simulink model "PriceCalc"  (R2021b)
settings: Solver=VariableStepAuto  StartTime=0.0  StopTime=10.0  RelTol=1e-3
libraries: fuzblock x22, simulink x7
settings Model: Creator=nbelo  LastModifiedBy=nbelo
settings SolverCC: ZeroCrossControl=DisableAll

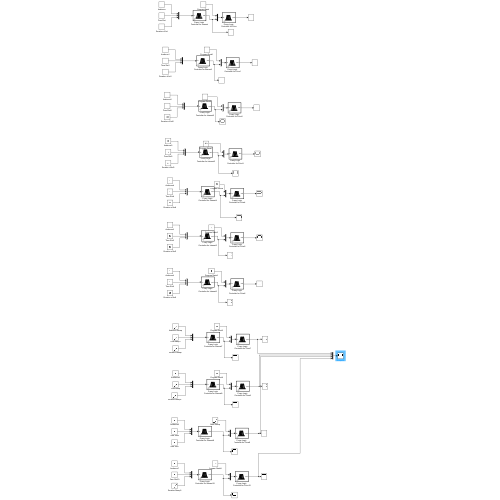
[thumbnail: Simulink's stored preview of the top-level diagram]
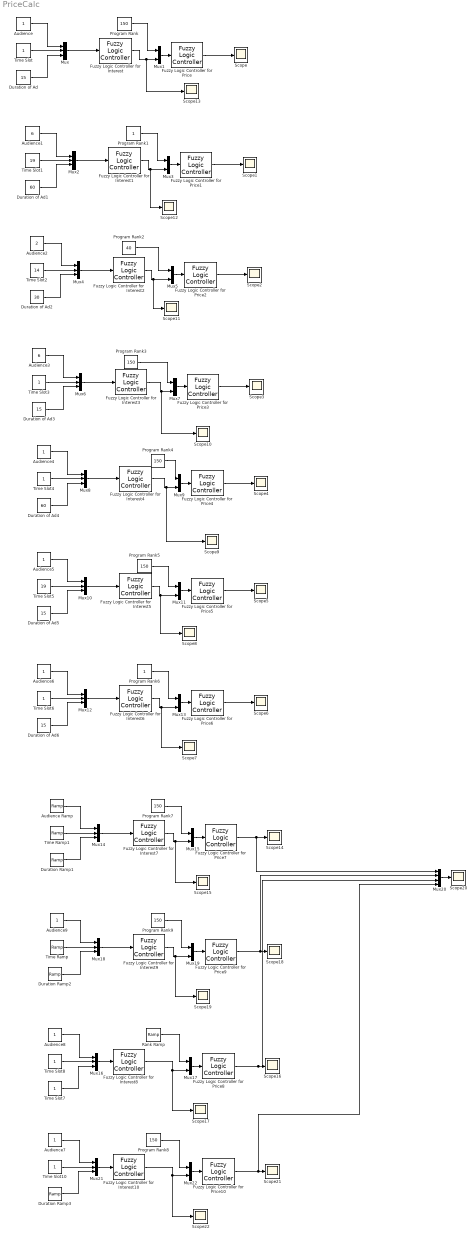
== system PriceCalc ==
  Audience{,4..9} (7 alike) : Constant
  Audience Ramp : simulink/Sources/Ramp  slope=.8  start=0  InitialOutput=0
  Audience1 : Constant  Value=6
  Audience2 : Constant  Value=2
  Audience3 : Constant  Value=6
  Duration Ramp1 : simulink/Sources/Ramp  slope=12  start=0  InitialOutput=0
  Duration Ramp2 : simulink/Sources/Ramp  slope=12  start=0  InitialOutput=0
  Duration Ramp3 : simulink/Sources/Ramp  slope=12  start=0  InitialOutput=0
  Duration of Ad{,3,5..6} (4 alike) : Constant  Value=15
  Duration of Ad1 : Constant  Value=60
  Duration of Ad2 : Constant  Value=30
  Duration of Ad4 : Constant  Value=60
  Fuzzy Logic Controller for Interest{,1..10} (11 alike) : fuzblock/Fuzzy Logic  Controller  FIS=Interest  OutputSampleNumber=101  DataType=double  FuzzifiedInputs=off  RuleFiringStrengths=off  RuleOutputs=off  AggregatedOutputs=off  SimulateUsing=Interpreted execution  OutOfRangeInputValueMessage=warning  NoRuleFiredMessage=warning  EmptyOutputFuzzySetMessage=warning
  Fuzzy Logic Controller for Price{,1..10} (11 alike) : fuzblock/Fuzzy Logic  Controller  FIS=Price  OutputSampleNumber=101  DataType=double  FuzzifiedInputs=off  RuleFiringStrengths=off  RuleOutputs=off  AggregatedOutputs=off  SimulateUsing=Interpreted execution  OutOfRangeInputValueMessage=warning  NoRuleFiredMessage=warning  EmptyOutputFuzzySetMessage=warning
  Mux{,2,4,6,8,10,12,14,16,18,21} (11 alike) : Mux  Inputs=3
  Mux{1,3,5,7,9,11,13,15,17,19,22} (11 alike) : Mux  Inputs=2
  Mux20 : Mux
  Program Rank{,3..5,7..9} (7 alike) : Constant  Value=150
  Program Rank1 : Constant
  Program Rank2 : Constant  Value=40
  Program Rank6 : Constant
  Rank Ramp : simulink/Sources/Ramp  slope=20  start=0  InitialOutput=0
  Scope{,1..22} (23 alike) : Scope
  Time Ramp : simulink/Sources/Ramp  slope=2.4  start=0  InitialOutput=0
  Time Ramp1 : simulink/Sources/Ramp  slope=2.4  start=0  InitialOutput=0
  Time Slot{,3..4,6..8,10} (7 alike) : Constant
  Time Slot1 : Constant  Value=19
  Time Slot2 : Constant  Value=14
  Time Slot5 : Constant  Value=19
  wires:
  Time Slot/1 -> Mux/2
  Audience/1 -> Mux/1
  Duration of Ad/1 -> Mux/3
  Mux/1 -> Fuzzy Logic Controller for Interest/1
  Mux1/1 -> Fuzzy Logic Controller for Price/1
  Fuzzy Logic Controller for Price/1 -> Scope/1
  Mux2/1 -> Fuzzy Logic Controller for Interest1/1
  Time Slot1/1 -> Mux2/2
  Audience1/1 -> Mux2/1
  Fuzzy Logic Controller for Price1/1 -> Scope1/1
  Mux3/1 -> Fuzzy Logic Controller for Price1/1
  Duration of Ad1/1 -> Mux2/3
  Mux4/1 -> Fuzzy Logic Controller for Interest2/1
  Time Slot2/1 -> Mux4/2
  Audience2/1 -> Mux4/1
  Fuzzy Logic Controller for Price2/1 -> Scope2/1
  Mux5/1 -> Fuzzy Logic Controller for Price2/1
  Duration of Ad2/1 -> Mux4/3
  Mux6/1 -> Fuzzy Logic Controller for Interest3/1
  Time Slot3/1 -> Mux6/2
  Audience3/1 -> Mux6/1
  Fuzzy Logic Controller for Price3/1 -> Scope3/1
  Mux7/1 -> Fuzzy Logic Controller for Price3/1
  Duration of Ad3/1 -> Mux6/3
  Mux8/1 -> Fuzzy Logic Controller for Interest4/1
  Time Slot4/1 -> Mux8/2
  Audience4/1 -> Mux8/1
  Fuzzy Logic Controller for Price4/1 -> Scope4/1
  Mux9/1 -> Fuzzy Logic Controller for Price4/1
  Duration of Ad4/1 -> Mux8/3
  Mux10/1 -> Fuzzy Logic Controller for Interest5/1
  Time Slot5/1 -> Mux10/2
  Audience5/1 -> Mux10/1
  Fuzzy Logic Controller for Price5/1 -> Scope5/1
  Mux11/1 -> Fuzzy Logic Controller for Price5/1
  Duration of Ad5/1 -> Mux10/3
  Mux12/1 -> Fuzzy Logic Controller for Interest6/1
  Time Slot6/1 -> Mux12/2
  Audience6/1 -> Mux12/1
  Fuzzy Logic Controller for Price6/1 -> Scope6/1
  Mux13/1 -> Fuzzy Logic Controller for Price6/1
  Duration of Ad6/1 -> Mux12/3
  Program Rank/1 -> Mux1/1
  Program Rank1/1 -> Mux3/1
  Fuzzy Logic Controller for Interest1/1 -> Scope12/1, Mux3/2
  Program Rank2/1 -> Mux5/1
  Fuzzy Logic Controller for Interest2/1 -> Scope11/1, Mux5/2
  Fuzzy Logic Controller for Interest3/1 -> Scope10/1, Mux7/2
  Program Rank3/1 -> Mux7/1
  Fuzzy Logic Controller for Interest4/1 -> Scope9/1, Mux9/2
  Program Rank4/1 -> Mux9/1
  Program Rank5/1 -> Mux11/1
  Fuzzy Logic Controller for Interest5/1 -> Scope8/1, Mux11/2
  Program Rank6/1 -> Mux13/1
  Fuzzy Logic Controller for Interest6/1 -> Scope7/1, Mux13/2
  Fuzzy Logic Controller for Interest/1 -> Scope13/1, Mux1/2
  Program Rank7/1 -> Mux15/1
  Fuzzy Logic Controller for Interest7/1 -> Scope15/1, Mux15/2
  Audience Ramp/1 -> Mux14/1
  Duration Ramp1/1 -> Mux14/3
  Mux14/1 -> Fuzzy Logic Controller for Interest7/1
  Time Ramp1/1 -> Mux14/2
  Fuzzy Logic Controller for Price7/1 -> Mux20/1, Scope14/1
  Mux15/1 -> Fuzzy Logic Controller for Price7/1
  Rank Ramp/1 -> Mux17/1
  Fuzzy Logic Controller for Interest8/1 -> Scope17/1, Mux17/2
  Time Slot7/1 -> Mux16/3
  Mux16/1 -> Fuzzy Logic Controller for Interest8/1
  Time Slot8/1 -> Mux16/2
  Fuzzy Logic Controller for Price8/1 -> Mux20/3, Scope16/1
  Mux17/1 -> Fuzzy Logic Controller for Price8/1
  Program Rank9/1 -> Mux19/1
  Fuzzy Logic Controller for Interest9/1 -> Scope19/1, Mux19/2
  Audience9/1 -> Mux18/1
  Duration Ramp2/1 -> Mux18/3
  Mux18/1 -> Fuzzy Logic Controller for Interest9/1
  Fuzzy Logic Controller for Price9/1 -> Mux20/2, Scope18/1
  Mux19/1 -> Fuzzy Logic Controller for Price9/1
  Mux20/1 -> Scope20/1
  Time Ramp/1 -> Mux18/2
  Audience8/1 -> Mux16/1
  Duration Ramp3/1 -> Mux21/3
  Mux22/1 -> Fuzzy Logic Controller for Price10/1
  Time Slot10/1 -> Mux21/2
  Mux21/1 -> Fuzzy Logic Controller for Interest10/1
  Fuzzy Logic Controller for Interest10/1 -> Scope22/1, Mux22/2
  Program Rank8/1 -> Mux22/1
  Audience7/1 -> Mux21/1
  Fuzzy Logic Controller for Price10/1 -> Mux20/4, Scope21/1
